simulink model "saturation_mask"  (R2021a)
settings: Solver=VariableStepAuto  StartTime=0.0  StopTime=10.0  RelTol=1e-3
settings Model: Creator=reemb  LastModifiedBy=reemb

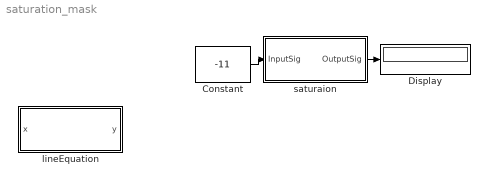
== system saturation_mask ==
  Constant : Constant  Value=-11
  Display : Display
  lineEquation : Subsystem  mask{m=10, b=3}
      mask prompts: m "slope"; b "intersection"
      mask DialogControl DescGroupVar Prompt: this block is model for line equation
      mask Display:
      | x=linspace(0,1,101);
      | t=linspace(0,1,101);
      | plot(x,t);
  saturaion : Subsystem  mask{upperlimit=10, lowerlimit=-10}
      mask prompts: upperlimit "upper limit"; lowerlimit "lower limit"
  wires:
  saturaion/1(OutputSig) -> Display/1
  Constant/1 -> saturaion/1(InputSig)

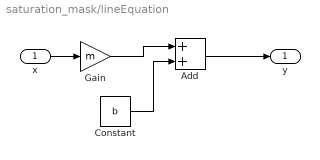
== system saturation_mask/lineEquation ==
  x : Inport
  Add : Sum
  Constant : Constant  Value=b
  Gain : Gain  Gain=m
  y : Outport
  wires:
  x/1 -> Gain/1
  Gain/1 -> Add/1
  Add/1 -> y/1
  Constant/1 -> Add/2

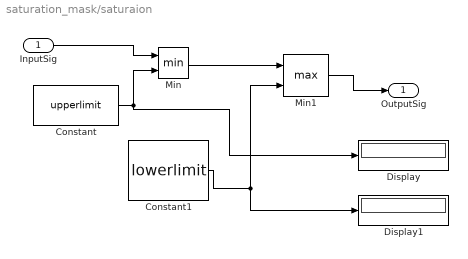
== system saturation_mask/saturaion ==
  InputSig : Inport
  Constant : Constant  Value=upperlimit
  Constant1 : Constant  Value=lowerlimit
  Display : Display
  Display1 : Display
  Min : MinMax  Inputs=2
  Min1 : MinMax  Function=max  Inputs=2
  OutputSig : Outport
  wires:
  InputSig/1 -> Min/1
  Min1/1 -> OutputSig/1
  Constant/1 -> Min/2, Display/1
  Constant1/1 -> Min1/2, Display1/1
  Min/1 -> Min1/1
